simulink model "ultracap_converter_simplified_PI_control_v4"  (R2012b)
settings: Solver=ode45  StartTime=0.0  StopTime=1  FixedStep=TsampleSimulink  MaxStep=1e-6  RelTol=1e-3
values from neighbouring files (symbols this model uses):
  Ts = 1/fs    (= 0.0002)    [load_system_parameters.m]
  Ts2 = 1/fs2    (= 0.05)    [load_system_parameters.m]
  Vbat = 12.1    [load_system_parameters.m]    (also in me547_based_simulator_v1.m = 48)
undefined symbols (not defined in the file or in its folder): Ea, Kp_vc, plecs, Ra, tf_TWA, tf_TWA2, VUCcommand_z
libraries: dspsigops x3, simulink x1
settings Model: Creator=Raghav  LastModifiedBy=Raghav

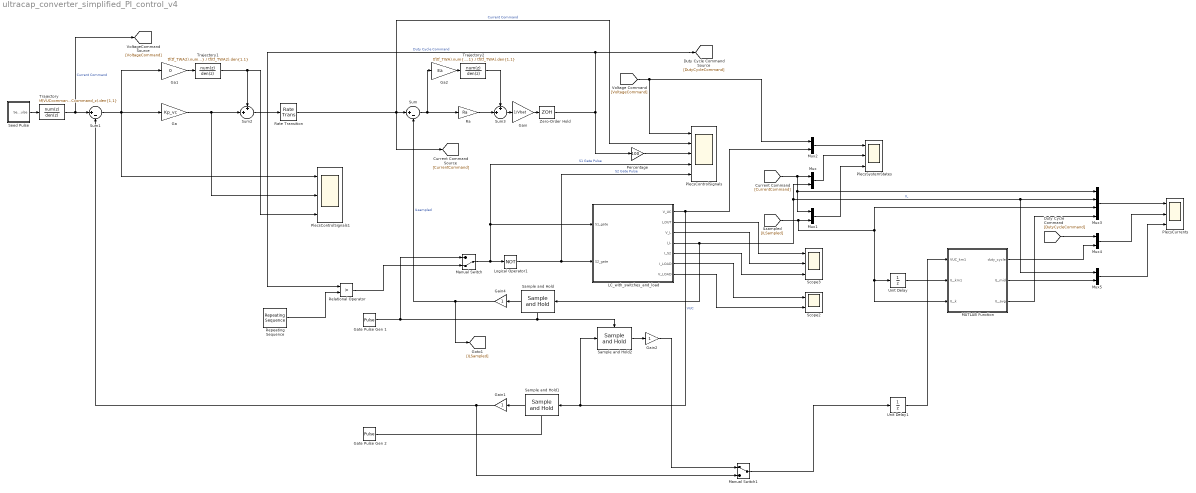
== system ultracap_converter_simplified_PI_control_v4 ==
  Ga : Gain  Gain=Kp_vc  SampleTime=Ts2
  Ga1 : Gain  Gain=0  SampleTime=Ts2
  Ga2 : Gain  Gain=Ea  SampleTime=Ts
  Gain : Gain  Gain=1/Vbat
  Gain1 : Gain  SampleTime=Ts2
  Gain2 : Gain  SampleTime=Ts
  Gain4 : Gain  SampleTime=Ts
  Gate Pulse Gen 1 : DiscretePulseGenerator  PulseType=Time based  Period=Ts  PulseWidth=0.1
  Gate Pulse Gen 2 : DiscretePulseGenerator  PulseType=Time based  Period=Ts2  PulseWidth=0.1
  LC_with_switches_and_load : Subsystem  LoadFcn=plecs('sl', 200);  InitFcn=plecs('sl', 214);  StartFcn=plecs('sl', 208);  StopFcn=plecs('sl', 209);  mask(PlecsCircuit){PLECSData=<binary blob, 2108 chars, not shown>}
      mask prompts: PLECSData "PLECS Data (Do not delete or modify!)"
      mask init:
      | % PLACE CUSTOM INITIALIZATIONS ABOVE
      | % DO NOT REMOVE
      | plecs('sl', 215);
      | % DO NOT REMOVE
      settings: CopyFcn=plecs('sl', 203);  DeleteFcn=plecs('sl', 205);  UndoDeleteFcn=plecs('sl', 206);  PreSaveFcn=plecs('sl', 211);  PostSaveFcn=plecs('sl', 201);  NameChangeFcn=plecs('sl', 210);  DestroyFcn=plecs('sl', 207);  PreCopyFcn=plecs('sl', 216);  OpenFcn=plecs('sl', 202);  ErrorFcn=plerrorfcn
      mask Help: web(['file:///' fullfile(plecsdoc, 'creatingacircuit.html')])
      mask Display: disp('PLECS\nCircuit')
  Logical Operator1 : Logic  Operator=NOT  AllPortsSameDT=off  OutDataTypeStr=boolean
  MATLAB Function : MATLAB Function  TreatAsAtomicUnit=on
  Manual Switch : ManualSwitch  CurrentSetting=0
  Manual Switch1 : ManualSwitch
  Mux{,1..2,4..5} (5 alike) : Mux  Inputs=2
  Mux3 : Mux
  Percentage : Gain  Gain=100
  PlecsControlSignals : Scope  NumInputPorts=5
      settings: TimeRange=2  YMin=0~0~-50~0~0  YMax=5~400~100~1~1  SaveName=PlecsControlSignals
  PlecsControlSignals1 : Scope  NumInputPorts=3
      settings: TimeRange=2  YMin=-100~-5~-5  YMax=300~5~5  SaveName=PlecsControlSignals1
  PlecsCurrents : Scope  NumInputPorts=3
      settings: ShowLegends=on  YMin=245~25~25  YMax=260~350~350  SaveName=PlecsCurrents
  PlecsSystemStates : Scope  NumInputPorts=3
      settings: ShowLegends=on  YMin=245~25~25  YMax=260~350~350  SaveName=PlecsSystemStates
  Ra : Gain  Gain=Ra  SampleTime=Ts
  Rate Transition : RateTransition  OutPortSampleTime=Ts
  Relational Operator : RelationalOperator  Priority=50  Operator=>  OutDataTypeStr=boolean
  Repeating Sequence : simulink/Sources/Repeating Sequence  rep_seq_t=[0 Ts]  rep_seq_y=[0 1]
  Sample and Hold : dspsigops/Sample and Hold  trig=Rising edge  initCond=0  latchinput=on
  Sample and Hold1 : dspsigops/Sample and Hold  trig=Rising edge  initCond=0  latchinput=on
  Sample and Hold2 : dspsigops/Sample and Hold  trig=Rising edge  initCond=0  latchinput=on
  Scope2 : Scope  NumInputPorts=2
      settings: ShowLegends=on  YMin=-5~-5  YMax=5~5  SaveName=ScopeData2
  Scope3 : Scope  NumInputPorts=3
      settings: ShowLegends=on  YMin=0~-50~-5  YMax=3.75~650~5  SaveName=Scope3
  Seed Pulse : Subsystem
  Sum : Sum  Inputs=|+-
  Sum1 : Sum  Inputs=|+-
  Sum2 : Sum  Inputs=++|
  Sum3 : Sum  Inputs=++|
  Trajectory : DiscreteTransferFcn  Numerator=tf(VUCcommand_z).num{1,1}  Denominator=tf(VUCcommand_z).den{1,1}  SampleTime=Ts2
  Trajectory1 : DiscreteTransferFcn  Numerator=tf(tf_TWA2).num{1,1}  Denominator=tf(tf_TWA2).den{1,1}  SampleTime=Ts2
  Trajectory2 : DiscreteTransferFcn  Numerator=tf(tf_TWA).num{1,1}  Denominator=tf(tf_TWA).den{1,1}  SampleTime=Ts
  Unit Delay : UnitDelay  SampleTime=-1
  Unit Delay1 : UnitDelay  SampleTime=-1
  Zero-Order Hold : ZeroOrderHold  SampleTime=Ts
  wires:
  LC_with_switches_and_load/1(V_UC) -> Mux2/2, Sample and Hold2/1, Sample and Hold1/1  "VUC"
  LC_with_switches_and_load/7(V_LOAD) -> Scope2/2
  LC_with_switches_and_load/4(I_L) -> Mux/2, Mux5/1, Mux3/2, Sample and Hold/1  "IL"
  LC_with_switches_and_load/6(I_LOAD) -> Scope2/1
  Logical Operator1/1 -> PlecsControlSignals/5, LC_with_switches_and_load/2(S2_gate)  "S2 Gate Pulse"
  Manual Switch/1 -> Logical Operator1/1, LC_with_switches_and_load/1(S1_gate), PlecsControlSignals/4  "S1 Gate Pulse"
  Seed Pulse/1(Seed Pulse) -> Trajectory/1
  Rate Transition/1 -> [CurrentCommand], PlecsControlSignals/2, Sum/1  "Current Command"
  Ra/1 -> Sum3/2
  Zero-Order Hold/1 -> [DutyCycleCommand], Relational Operator/1, Percentage/1  "Duty Cycle Command"
  Repeating Sequence/1 -> Relational Operator/2
  Gain/1 -> Zero-Order Hold/1
  Gate Pulse Gen 1/1 -> Manual Switch/1, Sample and Hold2/Trigger, Sample and Hold/Trigger
  Relational Operator/1 -> Manual Switch/2
  Sample and Hold/1 -> Gain4/1
  Gain4/1 -> [ILSampled], Sum/2  "ILsampled"
  LC_with_switches_and_load/2(I_OUT) -> Scope3/1
  LC_with_switches_and_load/3(V_L) -> Scope3/2
  LC_with_switches_and_load/5(I_S2) -> Scope3/3
  [CurrentCommand] -> Mux1/1, Mux3/1, Mux/1
  Mux/1 -> PlecsSystemStates/2
  Mux1/1 -> PlecsSystemStates/3
  [ILSampled] -> MATLAB Function/3(IL_k), Unit Delay/1, Mux3/3, Mux1/2
  Percentage/1 -> PlecsControlSignals/3
  Gate Pulse Gen 2/1 -> Sample and Hold1/Trigger
  Sample and Hold1/1 -> Gain1/1
  Trajectory/1 -> [VoltageCommand], Sum1/1  "Current Command"
  Gain1/1 -> Manual Switch1/2, Sum1/2
  Sum1/1 -> PlecsControlSignals1/1, Ga1/1, Ga/1
  [VoltageCommand] -> Mux2/1, PlecsControlSignals/1
  Mux2/1 -> PlecsSystemStates/1
  Mux3/1 -> PlecsCurrents/1
  Sample and Hold2/1 -> Gain2/1
  Gain2/1 -> Manual Switch1/1
  Manual Switch1/1 -> Unit Delay1/1
  Unit Delay/1 -> MATLAB Function/2(IL_km1)
  MATLAB Function/3(IL_avg) -> Mux3/4
  [DutyCycleCommand] -> Mux4/1
  MATLAB Function/1(duty_cycle) -> Mux4/2
  Mux4/1 -> PlecsCurrents/2
  MATLAB Function/2(IL_mid) -> Mux5/2
  Mux5/1 -> PlecsCurrents/3
  Unit Delay1/1 -> MATLAB Function/1(VUC_km1)
  Ga1/1 -> Trajectory1/1
  Ga/1 -> PlecsControlSignals1/2, Sum2/2
  Sum2/1 -> Rate Transition/1
  Trajectory1/1 -> Sum2/1, PlecsControlSignals1/3
  Sum/1 -> Ga2/1, Ra/1
  Trajectory2/1 -> Sum3/1
  Ga2/1 -> Trajectory2/1
  Sum3/1 -> Gain/1

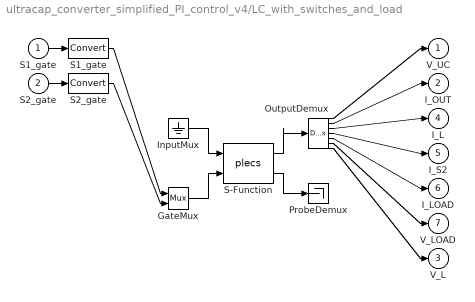
== system ultracap_converter_simplified_PI_control_v4/LC_with_switches_and_load ==
  S1_gate : Inport  PortDimensions=1
  S2_gate : Inport  Port=2  PortDimensions=1
  " GateMux " : Mux  Inputs=[ 1 1 ]
  " InputMux " : Ground
  " OutputDemux " : Demux  Outputs=[ 1 1 1 1 1 1 1 ]
  " ProbeDemux " : Terminator
  " S-Function " : S-Function  FunctionName=plecs  EnableBusSupport=off
  " S1_gate " : DataTypeConversion  SaturateOnIntegerOverflow=on  RndMeth=Zero
  " S2_gate " : DataTypeConversion  SaturateOnIntegerOverflow=on  RndMeth=Zero
  V_UC : Outport  PortDimensions=1
  I_OUT : Outport  Port=2  PortDimensions=1
  V_L : Outport  Port=3  PortDimensions=1
  I_L : Outport  Port=4  PortDimensions=1
  I_S2 : Outport  Port=5  PortDimensions=1
  I_LOAD : Outport  Port=6  PortDimensions=1
  V_LOAD : Outport  Port=7  PortDimensions=1
  wires:
  " S-Function "/2 -> " ProbeDemux "/1
  " GateMux "/1 -> " S-Function "/2
  " InputMux "/1 -> " S-Function "/1
  " S-Function "/1 -> " OutputDemux "/1
  S1_gate/1 -> " S1_gate "/1
  " S1_gate "/1 -> " GateMux "/1
  S2_gate/1 -> " S2_gate "/1
  " S2_gate "/1 -> " GateMux "/2
  " OutputDemux "/1 -> V_UC/1
  " OutputDemux "/2 -> I_OUT/1
  " OutputDemux "/3 -> I_L/1
  " OutputDemux "/4 -> I_S2/1
  " OutputDemux "/5 -> I_LOAD/1
  " OutputDemux "/6 -> V_LOAD/1
  " OutputDemux "/7 -> V_L/1

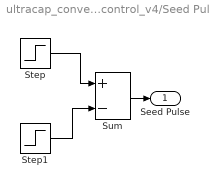
== system ultracap_converter_simplified_PI_control_v4/Seed Pulse ==
  Step : Step  Time=Ts2  SampleTime=0
  Step1 : Step  Time=Ts2+Ts2/2  SampleTime=0
  Sum : Sum  Inputs=+-
  Seed Pulse : Outport
  wires:
  Sum/1 -> Seed Pulse/1
  Step/1 -> Sum/1
  Step1/1 -> Sum/2

== matlab function ultracap_converter_simplified_PI_control_v4/MATLAB Function ==
  data: VUC_km1 input; duty_cycle output; IL_km1 input; IL_k input; IL_mid output; IL_avg output
function [duty_cycle, IL_mid, IL_avg] = fcn(VUC_km1, IL_km1, IL_k)

Vbat = 350;
L = 195e-6;
C = 30;
R = 3.6e-3 + 30e-3;
% R = 3.6e-3;
fs = 20e3;
Ts = 1/fs;
TsampleSimulink = Ts*1e-4;

del = R/2*sqrt(C/L);
w_r = 1/sqrt(L*C);

%#codegen

A = [   -(Vbat-VUC_km1)*w_r^2*C*Ts              1           ;
        VUC_km1*w_r^2*C*Ts                      1           ];
    
B = [   IL_km1                      ;
        IL_k+VUC_km1*w_r^2*C*Ts     ];
    
% now solve linear equation

X = A\B;

duty_cycle = X(1);
IL_mid = X(2);

IL_avg = 0.5 * ( IL_mid + duty_cycle*IL_km1 + (1-duty_cycle)*IL_k );
